simulink model "SIL_Raspi_control_panel"  (R2018b)
settings: Solver=VariableStepAuto  StartTime=0.0  StopTime=30  RelTol=1e-3  EnableMultiTasking=on
values from neighbouring files (symbols this model uses):
  INTAB1 = INTAB{1}    [MVP4.m]
  INTAB3 = INTAB{3}    [MVP4.m]
  INTAB4 = zeros(length(height), 6)    [MVP4.m]
libraries: embdlinuxlib x2, raspberrypilib x1
settings Model: ExtModeTrigDuration=2  Creator=benkl  LastModifiedBy=benkl
settings SolverCC: PositivePriorityOrder=on  AutoInsertRateTranBlk=on
settings OptimizationCC: EnhancedBackFolding=on  PassReuseOutputArgsAs=Individual arguments  MaxStackSize=64  OptimizeBlockOrder=speed  DifferentSizesBufferReuse=on  OptimizationCustomize=off
settings DebuggingCC: ParameterTunabilityLossMsg=error
settings HardwareCC: ProdBitPerPointer=32  ProdBitPerSizeT=32  ProdBitPerPtrDiffT=32  ProdLargestAtomicInteger=Long  ProdLargestAtomicFloat=Double  ProdWordSize=32  ProdHWDeviceType=ARM Compatible->ARM Cortex
settings SFSimCC: MATLABDynamicMemAlloc=off
settings RTWCC: SystemTargetFile=ert.tlc  HardwareBoard=Raspberry Pi  TLCOptions="-aInlineSetEventsForThisBaseRateFcn=TLC_FALSE -aSuppressMultiTaskScheduler=TLC_FALSE  -aRateBasedStepFcn=0"  TemplateMakefile=ert_default_tmf  Toolchain=GNU GCC Raspberry Pi  BuildConfiguration=Faster Runs  IncludeHyperlinkInReport=on
settings CodeAppCC: ForceParamTrailComments=on  IgnoreCustomStorageClasses=off  OperatorAnnotations=on  SimulinkDataObjDesc=on  SFDataObjDesc=on  InsertBlockDesc=on
settings ERTTargetCC: SupportContinuousTime=on  SupportVariableSizeSignals=on  ExtMode=on  ExtModeMexArgs='192.168.137.74' 0 17725

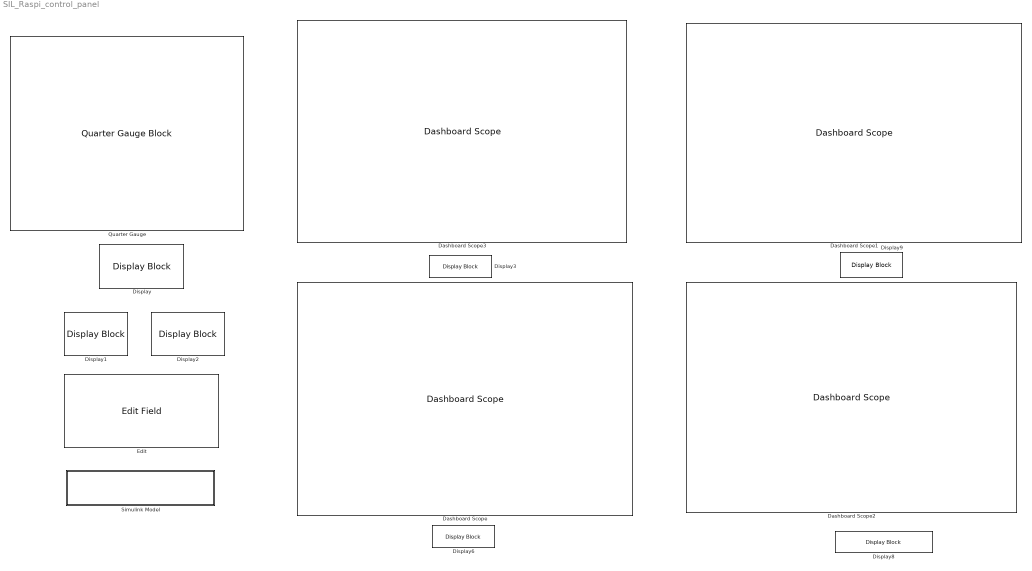
== system SIL_Raspi_control_panel ==
  Dashboard Scope : DashboardScope  WebBlockId=367  Ymin=0  Ymax=400
  Dashboard Scope1 : DashboardScope  WebBlockId=368  Ymin=0  Ymax=4000
  Dashboard Scope2 : DashboardScope  WebBlockId=406  Ymin=0.0030000000000000001  Ymax=0.01  ScaleAtStop=off
  Dashboard Scope3 : DashboardScope  WebBlockId=376  Ymin=-0.5  Ymax=0.5  ScaleAtStop=off
  Display : DisplayBlock  WebBlockId=375
  Display1 : DisplayBlock  WebBlockId=377
  Display2 : DisplayBlock  WebBlockId=379
  Display3 : DisplayBlock  WebBlockId=390  LabelPosition=Hide
  Display6 : DisplayBlock  WebBlockId=393  LabelPosition=Hide
  Display8 : DisplayBlock  WebBlockId=395  LabelPosition=Hide
  Display9 : DisplayBlock  WebBlockId=396  LabelPosition=Hide
  Edit : EditField  WebBlockId=389  ShowInitialText=on  Alignment=Center
  Quarter Gauge : QuarterGaugeBlock  WebBlockId=374  ScaleMax=77
  Simulink Model : Subsystem

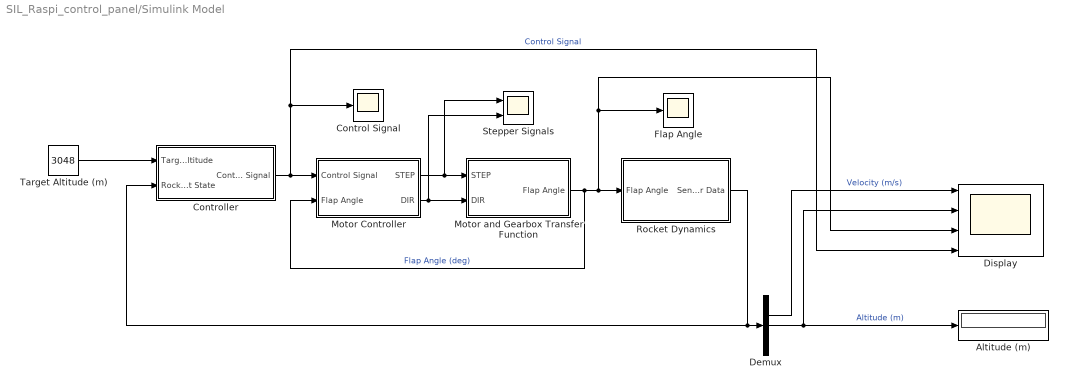
== system SIL_Raspi_control_panel/Simulink Model ==
  Altitude (m) : Display
  Control Signal : Scope
  Controller : Subsystem
  Demux : Demux  Outputs=5
  Display : Scope  NumInputPorts=4
  Flap Angle : Scope
  Motor Controller : Subsystem
  Motor and Gearbox Transfer Function : Subsystem
  Rocket Dynamics : Subsystem
  Stepper Signals : Scope  NumInputPorts=2
  "Target Altitude (m) " : Constant  Value=3048
  wires:
  Rocket Dynamics/1(Sensor Data) -> Demux/1, Controller/2(Rocket State)
  Motor and Gearbox Transfer Function/1(Flap Angle) -> Motor Controller/2(Flap Angle), Rocket Dynamics/1(Flap Angle), Display/3, Flap Angle/1  "Flap Angle (deg)"
  "Target Altitude (m) "/1 -> Controller/1(Target Altitude)
  Controller/1(Control Signal) -> Display/4, Control Signal/1, Motor Controller/1(Control Signal)  "Control Signal"
  Motor Controller/2(DIR) -> Stepper Signals/2, Motor and Gearbox Transfer Function/2(DIR)
  Motor Controller/1(STEP) -> Stepper Signals/1, Motor and Gearbox Transfer Function/1(STEP)
  Demux/2 -> Display/1  "Velocity (m/s)"
  Demux/3 -> Altitude (m)/1, Display/2  "Altitude (m)"

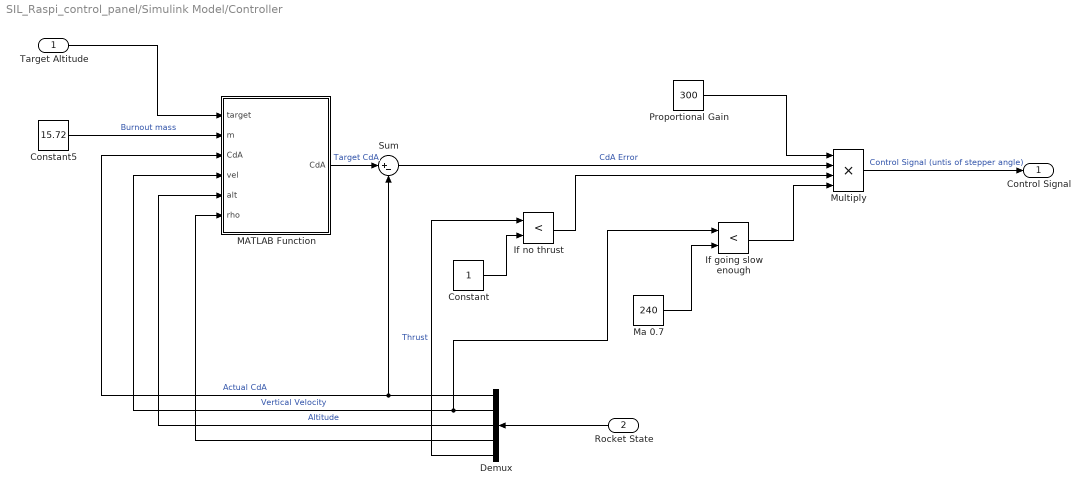
== system SIL_Raspi_control_panel/Simulink Model/Controller ==
  Target Altitude : Inport
  Rocket State : Inport  Port=2
  Constant : Constant
  Constant5 : Constant  Value=15.72
  Demux : Demux  Outputs=5
  If going slow enough : RelationalOperator  Operator=<  OutDataTypeStr=boolean  RndMeth=Simplest
  If no thrust : RelationalOperator  Operator=<  OutDataTypeStr=boolean  RndMeth=Simplest
  MATLAB Function : MATLAB Function  TreatAsAtomicUnit=on
  Ma 0.7 : Constant  Value=240
  Multiply : Product  Inputs=4
  Proportional Gain : Constant  Value=300
  Sum : Sum  Inputs=|+-
  Control Signal : Outport
  wires:
  Proportional Gain/1 -> Multiply/1
  Constant5/1 -> MATLAB Function/2(m)  "Burnout mass"
  Multiply/1 -> Control Signal/1  "Control Signal (untis of stepper angle)"
  MATLAB Function/1(CdA) -> Sum/1  "Target CdA"
  Sum/1 -> Multiply/2  "CdA Error"
  Demux/5 -> If no thrust/1  "Thrust"
  Rocket State/1 -> Demux/1
  Demux/3 -> MATLAB Function/5(alt)  "Altitude"
  Demux/2 -> If going slow enough/1, MATLAB Function/4(vel)  "Vertical Velocity"
  Demux/4 -> MATLAB Function/6(rho)
  Target Altitude/1 -> MATLAB Function/1(target)
  Demux/1 -> Sum/2, MATLAB Function/3("CdA ")  "Actual CdA"
  If no thrust/1 -> Multiply/3
  Constant/1 -> If no thrust/2
  If going slow enough/1 -> Multiply/4
  Ma 0.7/1 -> If going slow enough/2

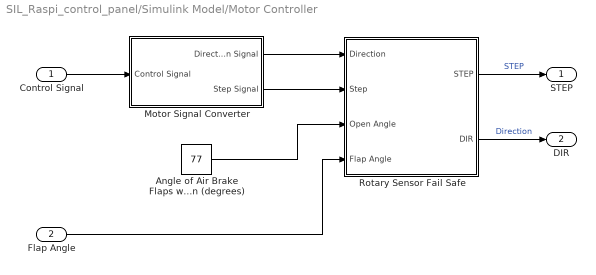
== system SIL_Raspi_control_panel/Simulink Model/Motor Controller ==
  Control Signal : Inport
  Flap Angle : Inport  Port=2
  Angle of Air Brake Flaps when Fully Open (degrees) : Constant  Value=77
  Motor Signal Converter : Subsystem
  Rotary Sensor Fail Safe : Subsystem
  STEP : Outport
  DIR : Outport  Port=2
  wires:
  Control Signal/1 -> Motor Signal Converter/1(Control Signal)
  Motor Signal Converter/2(Step Signal) -> Rotary Sensor Fail Safe/2(Step)
  Motor Signal Converter/1(Direction Signal) -> Rotary Sensor Fail Safe/1(Direction)
  Angle of Air Brake Flaps when Fully Open (degrees)/1 -> Rotary Sensor Fail Safe/3(Open Angle)
  Rotary Sensor Fail Safe/1(STEP) -> STEP/1  "STEP"
  Flap Angle/1 -> Rotary Sensor Fail Safe/4(Flap Angle)
  Rotary Sensor Fail Safe/2(DIR) -> DIR/1  "Direction"

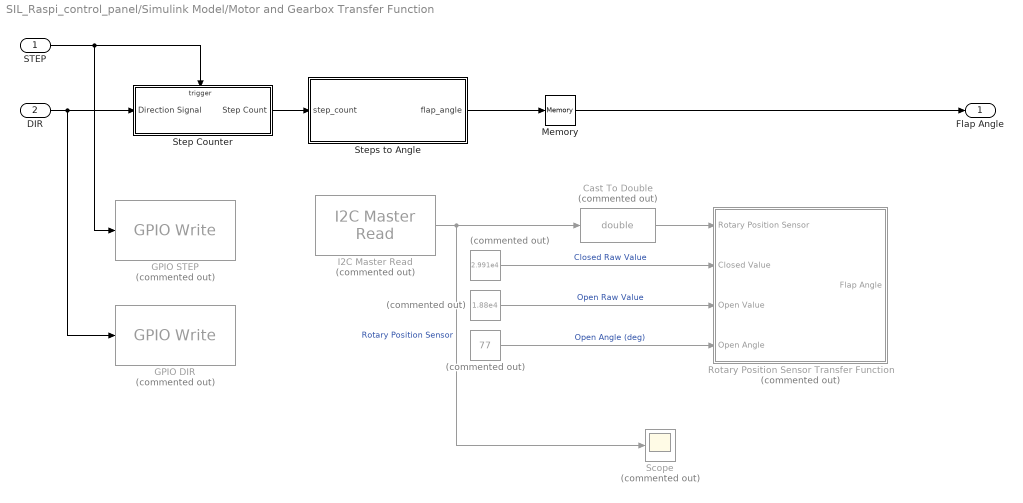
== system SIL_Raspi_control_panel/Simulink Model/Motor and Gearbox Transfer Function ==
  STEP : Inport
  DIR : Inport  Port=2
  " " : Constant  Commented=on  Value=2.991e4
  "  " : Constant  Commented=on  Value=77
  " " : Constant  Commented=on  Value=1.88e4
  Cast To Double : DataTypeConversion  Commented=on  OutDataTypeStr=double
  GPIO DIR : embdlinuxlib/GPIO Write  Commented=on  board=Model B+  gpio=21  direction=Output  blockPlatform=Raspberry Pi
      settings: SourceProductName=Simulink Support Package for Raspberry Pi Hardware  SourceProductBaseCode=RASPPI
  GPIO STEP : embdlinuxlib/GPIO Write  Commented=on  board=Model B+  gpio=20  direction=Output  blockPlatform=Raspberry Pi
      settings: SourceProductName=Simulink Support Package for Raspberry Pi Hardware  SourceProductBaseCode=RASPPI
  I2C Master Read : raspberrypilib/I2C Master Read  Commented=on  BoardProperty=Pi 3 Model B+  Mode=Master  SlaveAddress=72  SlaveByteOrder=BigEndian  Direction=Receiver  RegisterAddressMode=on  RegisterAddress=0  SlaveDataType=int16  DataLength=1  NoAck=off  RepeatedStart=off  OutputStatus=off  SampleTime=0.005
      settings: SourceProductName=Simulink Support Package for Raspberry Pi Hardware  SourceProductBaseCode=RASPPI
  Memory : Memory
  Rotary Position Sensor Transfer Function : Subsystem  Commented=on
  Scope : Scope  Commented=on
  Step Counter : Subsystem
  Steps to Angle : MATLAB Function  TreatAsAtomicUnit=on
  Flap Angle : Outport
  wires:
  Step Counter/1(Step Count) -> Steps to Angle/1(step_count)
  Steps to Angle/1(flap_angle) -> Memory/1
  "  "/1 -> Rotary Position Sensor Transfer Function/4(Open Angle)  "Open Angle (deg)"
  I2C Master Read/1 -> Scope/1, Cast To Double/1  "Rotary Position Sensor"
  " "/1 -> Rotary Position Sensor Transfer Function/2(Closed Value)  "Closed Raw Value"
  " "/1 -> Rotary Position Sensor Transfer Function/3(Open Value)  "Open Raw Value"
  STEP/1 -> GPIO STEP/1, Step Counter/Trigger
  DIR/1 -> GPIO DIR/1, Step Counter/1(Direction Signal)
  Cast To Double/1 -> Rotary Position Sensor Transfer Function/1(Rotary Position Sensor)
  Memory/1 -> Flap Angle/1

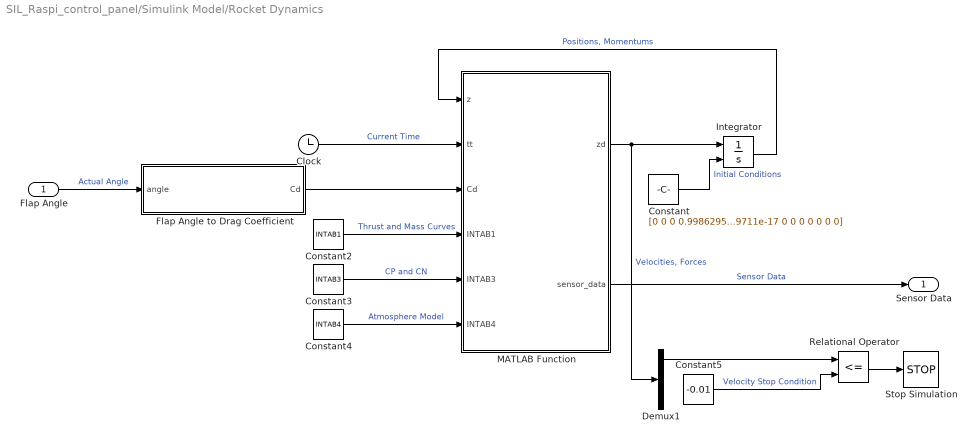
== system SIL_Raspi_control_panel/Simulink Model/Rocket Dynamics ==
  Flap Angle : Inport
  Clock : Clock
  Constant : Constant  Value="[0\t0\t0\t0.998629534754574\t-0.0523359562429438\t1.92279183879711e-17\t0\t0\t0\t0\t0\t0\t0]"
  Constant2 : Constant  Value=INTAB1  VectorParams1D=off
  Constant3 : Constant  Value=INTAB3  VectorParams1D=off
  Constant4 : Constant  Value=INTAB4  VectorParams1D=off
  Constant5 : Constant  Value=-0.01
  Demux1 : Demux  Outputs=13
  Flap Angle to Drag Coefficient : MATLAB Function  TreatAsAtomicUnit=on
  Integrator : Integrator  InitialConditionSource=external
  MATLAB Function : MATLAB Function  TreatAsAtomicUnit=on
  Relational Operator : RelationalOperator  Operator=<=  OutDataTypeStr=boolean  RndMeth=Simplest
  Stop Simulation : Stop
  Sensor Data : Outport
  wires:
  Clock/1 -> MATLAB Function/2(tt)  "Current Time"
  Integrator/1 -> MATLAB Function/1(z)  "Positions, Momentums"
  Constant4/1 -> MATLAB Function/6(INTAB4)  "Atmosphere Model"
  MATLAB Function/1(zd) -> Integrator/1, Demux1/1  "Velocities, Forces"
  Constant5/1 -> Relational Operator/2  "Velocity Stop Condition"
  Constant3/1 -> MATLAB Function/5(INTAB3)  "CP and CN"
  Constant2/1 -> MATLAB Function/4(INTAB1)  "Thrust and Mass Curves"
  MATLAB Function/2(sensor_data) -> Sensor Data/1  "Sensor Data"
  Flap Angle/1 -> Flap Angle to Drag Coefficient/1(angle)  "Actual Angle"
  Flap Angle to Drag Coefficient/1(Cd) -> MATLAB Function/3(Cd)
  Relational Operator/1 -> Stop Simulation/1
  Constant/1 -> Integrator/2  "Initial Conditions"
  Demux1/3 -> Relational Operator/1

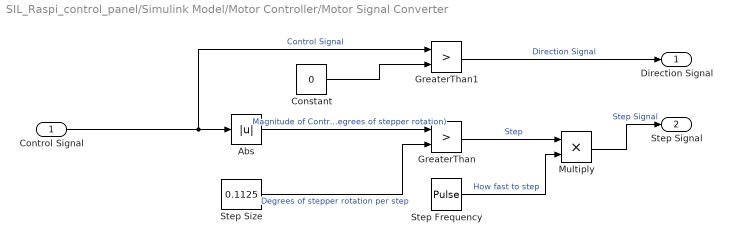
== system SIL_Raspi_control_panel/Simulink Model/Motor Controller/Motor Signal Converter ==
  Control Signal : Inport
  Abs : Abs
  Constant : Constant  Value=0
  GreaterThan : RelationalOperator  Operator=>  OutDataTypeStr=boolean  RndMeth=Simplest
  GreaterThan1 : RelationalOperator  Operator=>  OutDataTypeStr=boolean  RndMeth=Simplest
  Multiply : Product
  Step Frequency : DiscretePulseGenerator  PulseType=Time based  Period=0.005  PulseWidth=50
  Step Size : Constant  Value=0.1125
  Direction Signal : Outport
  Step Signal : Outport  Port=2
  wires:
  Abs/1 -> GreaterThan/1  "Magnitude of Control Signal (degrees of stepper rotation)"
  Constant/1 -> GreaterThan1/2
  Step Size/1 -> GreaterThan/2  "Degrees of stepper rotation per step"
  Control Signal/1 -> GreaterThan1/1, Abs/1  "Control Signal"
  Step Frequency/1 -> Multiply/2  "How fast to step"
  GreaterThan/1 -> Multiply/1  "Step"
  Multiply/1 -> Step Signal/1  "Step Signal"
  GreaterThan1/1 -> Direction Signal/1  "Direction Signal"

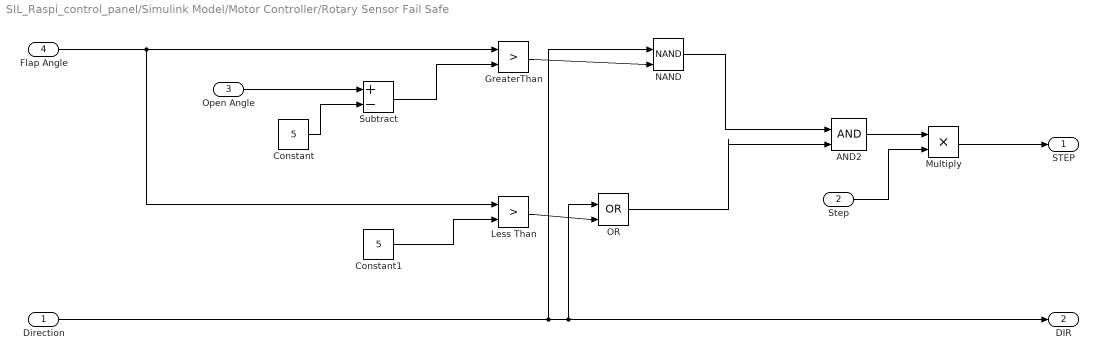
== system SIL_Raspi_control_panel/Simulink Model/Motor Controller/Rotary Sensor Fail Safe ==
  Direction : Inport
  Step : Inport  Port=2
  Open Angle : Inport  Port=3
  Flap Angle : Inport  Port=4
  AND2 : Logic  IconShape=distinctive  AllPortsSameDT=off  OutDataTypeStr=boolean
  Constant : Constant  Value=5
  Constant1 : Constant  Value=5
  GreaterThan : RelationalOperator  Operator=>  OutDataTypeStr=boolean  RndMeth=Simplest
  Less Than : RelationalOperator  Operator=>  OutDataTypeStr=boolean  RndMeth=Simplest
  Multiply : Product
  NAND : Logic  Operator=NAND  IconShape=distinctive  AllPortsSameDT=off  OutDataTypeStr=boolean
  OR : Logic  Operator=OR  IconShape=distinctive  AllPortsSameDT=off  OutDataTypeStr=boolean
  Subtract : Sum  Inputs=+-
  STEP : Outport
  DIR : Outport  Port=2
  wires:
  Flap Angle/1 -> Less Than/1, GreaterThan/1
  Constant/1 -> Subtract/2
  Open Angle/1 -> Subtract/1
  Subtract/1 -> GreaterThan/2
  GreaterThan/1 -> NAND/2
  Multiply/1 -> STEP/1
  Step/1 -> Multiply/2
  Direction/1 -> NAND/1, OR/1, DIR/1
  AND2/1 -> Multiply/1
  Less Than/1 -> OR/2
  Constant1/1 -> Less Than/2
  OR/1 -> AND2/2
  NAND/1 -> AND2/1

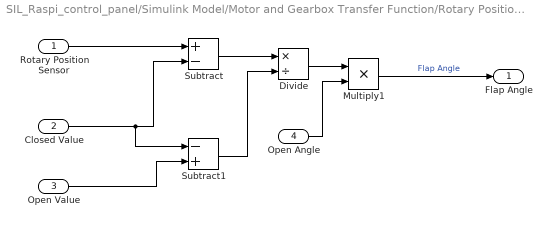
== system SIL_Raspi_control_panel/Simulink Model/Motor and Gearbox Transfer Function/Rotary Position Sensor Transfer Function ==
  Rotary Position Sensor : Inport
  Closed Value : Inport  Port=2
  Open Value : Inport  Port=3
  Open Angle : Inport  Port=4
  Divide : Product  Inputs=*/
  Multiply1 : Product
  Subtract : Sum  Inputs=+-
  Subtract1 : Sum  Inputs=-+
  Flap Angle : Outport
  wires:
  Subtract/1 -> Divide/1
  Closed Value/1 -> Subtract1/1, Subtract/2
  Divide/1 -> Multiply1/1
  Open Angle/1 -> Multiply1/2
  Subtract1/1 -> Divide/2
  Rotary Position Sensor/1 -> Subtract/1
  Open Value/1 -> Subtract1/2
  Multiply1/1 -> Flap Angle/1  "Flap Angle"

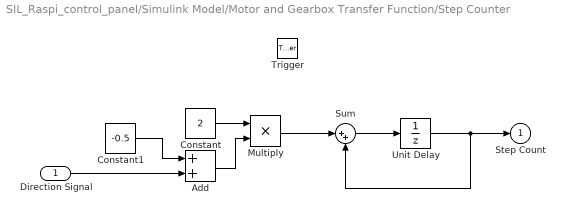
== system SIL_Raspi_control_panel/Simulink Model/Motor and Gearbox Transfer Function/Step Counter ==
  Direction Signal : Inport
  Trigger : TriggerPort  VariantControl=Variant  PortDimensions=1
  Add : Sum
  Constant : Constant  Value=2
  Constant1 : Constant  Value=-0.5
  Multiply : Product
  Sum : Sum  Inputs=|++  SaturateOnIntegerOverflow=on  InputSameDT=on  OutDataTypeStr=Inherit: Same as first input
  Unit Delay : UnitDelay  SampleTime=-1
  Step Count : Outport  InitialOutput=0
  wires:
  Direction Signal/1 -> Add/2
  Add/1 -> Multiply/2
  Constant1/1 -> Add/1
  Constant/1 -> Multiply/1
  Sum/1 -> Unit Delay/1
  Unit Delay/1 -> Step Count/1, Sum/2
  Multiply/1 -> Sum/1

== matlab function SIL_Raspi_control_panel/Simulink Model/Controller/MATLAB Function ==
  data: target input; m input; CdA output; CdA input; vel input; alt input; rho input
function CdA  = drag_predictor(target, m, CdA, vel, alt, rho)
%DRAG_PREDICTOR calculates the optimal drag coefficient based on current state

a = m/(rho*0.9); % bit of hard-coding jank to get the prediction more acurate
b = 2*9.81/vel^2;
c = target - alt;
CdA_opt = (-a*Lambert_W((-b*c*exp(-b*c)),-1)-a*b*c)/c; % Closed form solved in matlab

if isreal(CdA_opt) && ~isnan(CdA_opt)
%     if CdA_opt > 0.001 && CdA_opt < 0.01 % Set upper and lower bounds on CdA (m^2)
%         CdA = CdA_opt;
%     elseif CdA_opt < 0.001
%         CdA = 0.001;
%     else 
%         CdA = 0.01;
%     end
%     
    CdA = CdA_opt;
end

if alt > target % If already too high, put brakes on as much as possible
    CdA = 1;
end

    function w = Lambert_W(x,branch)
        % Lambert_W  Functional inverse of x = w*exp(w).
        % w = Lambert_W(x), same as Lambert_W(x,0)
        % w = Lambert_W(x,0)  Primary or upper branch, W_0(x)
        % w = Lambert_W(x,-1)  Lower branch, W_{-1}(x)
        %
        % See: https://blogs.mathworks.com/cleve/2013/09/02/the-lambert-w-function/

        % Copyright 2013 The MathWorks, Inc.

        % Effective starting guess
        if nargin < 2 || branch ~= -1
           w = ones(size(x));  % Start above -1
        else  
           w = -2*ones(size(x));  % Start below -1
        end
        v = inf*w;
        
        
        % Haley's method
        ii = 0;
        while any(abs(w - v)./abs(w) > 1.e-6) && ii<1000
           v = w;
           e = exp(w);
           f = w.*e - x;  % Iterate to make this quantity zero
           w = w - f./((e.*(w+1) - (w+2).*f./(2*w+2)));
           ii = ii+1;
        end
    end

% in.alt = alt; % [m] rocket's current altitude
% in.vel = vel; % [m/s] rocket's current velocity
% in.rho = rho; % [kg/m^3] density of air
% in.m = m; % [kg] mass of rocket after burnout
% 
% % options = optimset('TolX', 1e-7);
% % [CdA_opt,~,exitflag] = fzero(@apogeeerror, CdA, options);
% % 
% % if exitflag==1
% %     CdA = CdA_opt;
% % end
% % 
% % 
% % 
% %     function apogee = apogeeerror(CdA) % Finds the difference between the estimated and actual apogee
% %         x = log( complex(CdA*rho/(2*m*9.81)*vel^2 + 1) );
% %         if isreal(x)
% %             apogee = alt + m/(CdA*rho) * x - target;
% %         else
% %             apogee = 1e9;
% %         end
% %     end
% 
% % 
% % try
%     CdA_opt = secant(@apogeeerror, CdA, in); % Might want to use a more robust solver in the future
%     if CdA_opt > 0.001 && CdA_opt < 0.01 % Set upper and lower bounds on CdA (m^2)
%         CdA = CdA_opt;
%     end % Otherwise keep estimated term for CdA
% % catch
% % end
% %     
% 
%     function [x] = secant(fun, x1, in)
%     %SECANT is a zero-finding function based on the secant method
%     %   'fun' is the function handle for which the zero is desired
%     %   'x1' is the initial guess
%     %   'in' is a struct containing any additional inputs 'fun' might require
%     %   'x' is the value of the zero
%         x_eps = x1*0.005; % Set the tolerance to be 0.5% of initial guess
%         x2 = x1-x1*0.01; % Set a second point 1% away from the original guess
%         F1 = fun(x1, in); % Evaluate function at x1
%         F2 = fun(x2, in); % Evaluate function at x2
%         
%         
%         
%         kk = 1; % Set up counter
%         kk_max = 100;
%         while abs(x2-x1)>=x_eps && kk<kk_max % While error is too large and counter is less than max
%             x3 = x2 - F2*(x2-x1)/(F2-F1);
%             x1 = x2; % Move everything forward
%             x2 = x3;
%             F1 = F2;
%             F2 = fun(x2, in);
%             if ~isreal(F2) % If non-real
%                 x = NaN;
%                 return
%             end
%             kk = kk+1;
%         end
%         x = x2;
%     end
% 
%     function apogee = apogeeerror(CdA, in) % Finds the difference between the estimated and actual apogee
% %         if CdA*in.rho/(2*in.m*9.81) * in.vel^2 + 1 <= 0
% %             sup = 0;
% %         end
%         apogee = in.alt + in.m/(CdA*in.rho) * log( complex(CdA*in.rho/(2*in.m*9.81) * in.vel^2 + 1) ) - target;
%     end

end

== matlab function SIL_Raspi_control_panel/Simulink Model/Motor and Gearbox Transfer Function/Steps to Angle ==
  data: step_count input; flap_angle output
function flap_angle = Steps_to_Angle_TF(step_count)
% Calulates the flap angle based on the stepper commands
%   Will be replaced by physical system in prototype

GR = 2.5; % Gear ratio between stepper and flap
step_size = 0.1125; % [degrees] angle of one step of the stepper

flap_angle = step_count*step_size*GR;

== matlab function SIL_Raspi_control_panel/Simulink Model/Rocket Dynamics/Flap Angle to Drag Coefficient ==
  data: angle input; Cd output
function Cd = dragTF(angle) % Angle is the flap angle (as sensed by position sensor)

%%%%%%%%%%%%%% REPLACE THIS WITH BETTER MODEL BASED ON CFD %%%%%%%%%%%%%%%%
% Also add mach number dependency

Cd_rocket = 0.4; % Coefficient of drag of rocket
A_ref = 0.010751315458748; % [m^2] rocket reference area
Cd_flat_plate = 1.1; % From CFD

A_flat_plate = -3.953e-7*angle^2 + 8.737e-5*angle + 4.547e-5; % Calculate exposed area (quadratic fit from solidworks angle-area points)
Cd = Cd_rocket + Cd_flat_plate*A_flat_plate/A_ref; % Calculate Drag Coefficient

== matlab function SIL_Raspi_control_panel/Simulink Model/Rocket Dynamics/MATLAB Function ==
  data: z input; tt input; zd output; Cd input; INTAB1 input; INTAB3 input; INTAB4 input; sensor_data output
function [zd,sensor_data]=blastoff6dof(z,tt,Cd,INTAB1,INTAB3,INTAB4)
% % Constants **************************************************************
% RL=4.3; % Launch rail length
% Ar=0.010751315458748; % Rocket aerodynamic reference area
% 
% 
% % Unpack z ***************************************************************
% zn=z(1); % Postion vector
% Pz=z(2); % Translational momentum vector
% 
% % Gravity ****************************************************************
% g=6.6742E-11*5.9742E24/(6378100+zn)^2;
% 
% 
% % EXTRACT DATA FROM INPUT TABLES 1, 3, and 4 *****************************
% % INTAB1 *****************************************************************
% t=INTAB1(:,1); % Get time data from input table
% if tt<=t(1)
%     Ti = INTAB1(1,2);
%     Mi = INTAB1(1,3);
% elseif tt<t(end) % If time is within bounds of array
%     for ii = 2:length(t)
%         if tt <= t(ii) % Find first index that is larger than OF
%             break
%         end
%     end
%     T = INTAB1(:,2);
%     Ti = (tt-t(ii-1))/(t(ii)-t(ii-1))*(T(ii)-T(ii-1)) + T(ii); % Thrust-time data
%     M = INTAB1(:,3);
%     Mi = (tt-t(ii-1))/(t(ii)-t(ii-1))*(M(ii)-M(ii-1)) + M(ii); % Mass-time data
% else
%     Ti=INTAB1(end,2);
%     Mi=INTAB1(end,3);
% end
% 
% % INTAB4 *****************************************************************
% ztb=INTAB4(:,1); %Get altitude data from input table
% if zn<ztb(end) && zn>=ztb(1)
%     for ii = 2:length(ztb)
%         if zn <= ztb(ii) % Find first index that is larger than OF
%             break
%         end
%     end
%     RHO = INTAB4(:,5);
%     rho = (zn-ztb(ii-1))/(ztb(ii)-ztb(ii-1))*(RHO(ii)-RHO(ii-1)) + RHO(ii); % Atmospheric density
%     TEMP = INTAB4(:,5);
%     temp = (zn-ztb(ii-1))/(ztb(ii)-ztb(ii-1))*(TEMP(ii)-TEMP(ii-1)) + TEMP(ii); % Atmospheric temperature
%     Pressure = 287*rho*temp;%Atmospheric Pressure
% else % If outside of table bounds
%     temp=(-131.21+(0.00299*zn))+273.15; % Random atmosphere model???
%     Pressure=0.002488*(temp/216.6)^-11.388;
%     rho=Pressure/287*temp;
% end
% 
% 
% % Rocket Velocity Calculations *******************************************
% Vz=Pz./Mi; % Rocket earth relative velocity vector
% 
% % Force vector calculations **********************************************
% FA=Cd*0.5*rho*(Vz^2)*Ar; % Calculate axial aerodynamic force
% mg=Mi*g; % Gravity
% 
% % Output calculations ****************************************************
% % Calculate position derivatives (velocities relative to earth)
% zdot=Vz;
% 
% % Calculate translational momentum derivatives (forces)
% if Ti<=mg && zn<0.1 % If thrust is smaller than gravity and flight just began
%     Fz=0;
% else
%     Fz=Ti-FA-mg; % Z Force vector component
% end
% 
% %ODE output
% zd=zeros(2,1);
% zd(1)=zdot;
% zd(2)=Fz;
% 
% % Sensor output **********************************************************
% sensor_data=zeros(5,1);
% sensor_data(1) = Cd*Ar; % CdA
% sensor_data(2) = zdot; % Vertical Velocity
% sensor_data(3) = zn; % Altitude
% sensor_data(4) = rho; % Air Density
% sensor_data(5) = Ti; % Thrust
% 
% 
% Constants **************************************************************
RL=4.3; % Launch rail length
Ar=0.010751315458748; % Rocket aerodynamic reference area


% Unpack z ***************************************************************
xn=z(1); % Postion vector
yn=z(2); % "
zn=z(3); % "
s=z(4); % Quaternion scalar
vx=z(5); % Quaternion vector
vy=z(6); % "
vz=z(7); % "
Px=z(8); % Translational momentum vector
Py=z(9); % "
Pz=z(10); % "
Ltheta=z(11); % Rotational momentum vector
Lphi=z(12); % "
Lpsi=z(13); % "

xt=[xn;yn;zn]; % Rocket position vector
qt=[s vx vy vz]; % Rocket quaternion
Pt=[Px;Py;Pz]; % Rocket translational momentum vector
Lt=[Ltheta;Lphi;Lpsi]; % Rocket rotational momentum vector


% Gravity ****************************************************************
g=6.6742E-11*5.9742E24/(6378100+zn)^2;


% EXTRACT DATA FROM INPUT TABLES 1, 3, and 4 *****************************
% INTAB1 *****************************************************************
t=INTAB1(:,1); % Get time data from input table
if tt<=t(1)
    Ti=INTAB1(1,2);
    Mi=INTAB1(1,3);
    Ixxi=INTAB1(1,4);
    Iyyi=INTAB1(1,5);
    Izzi=INTAB1(1,6);
    Ixyi=INTAB1(1,7);
    Ixzi=INTAB1(1,8);
    Iyzi=INTAB1(1,9);
    Xcmi=INTAB1(1,10);
    Cda1=INTAB1(1,11);
elseif tt<t(end) && tt>=t(1) % If time is within bounds of array
    Ti=interp1(t,INTAB1(:,2),tt); % Thrust-time data
    Mi=interp1(t,INTAB1(:,3),tt); % Mass-time data
    Ixxi=interp1(t,INTAB1(:,4),tt); % Moments of inertia-time data
    Iyyi=interp1(t,INTAB1(:,5),tt); % "
    Izzi=interp1(t,INTAB1(:,6),tt); % "
    Ixyi=interp1(t,INTAB1(:,7),tt); % Products of inertia-time data
    Ixzi=interp1(t,INTAB1(:,8),tt); % "
    Iyzi=interp1(t,INTAB1(:,9),tt); % "
    Xcmi=interp1(t,INTAB1(:,10),tt); % Center of mass-time data
    Cda1=interp1(t,INTAB1(:,11),tt); % Thrust damping moment coefficient
else
    Ti=INTAB1(end,2);
    Mi=INTAB1(end,3);
    Ixxi=INTAB1(end,4);
    Iyyi=INTAB1(end,5);
    Izzi=INTAB1(end,6);
    Ixyi=INTAB1(end,7);
    Ixzi=INTAB1(end,8);
    Iyzi=INTAB1(end,9);
    Xcmi=INTAB1(end,10);
    Cda1=INTAB1(end,11);
end
Ibody=[Ixxi Ixyi Ixzi;Ixyi Iyyi Iyzi;Ixzi Iyzi Izzi]; % Inertia tensor

% INTAB3 *****************************************************************
Cn=INTAB3(1);
Cp=INTAB3(2);

% INTAB4 *****************************************************************
ztb=INTAB4(:,1); %Get altitude data from input table
if zn<ztb(end) && zn>=ztb(1)
    Wxi=interp1(ztb,INTAB4(:,2),zn);%Wind velocity vector
    Wyi=interp1(ztb,INTAB4(:,3),zn);%"
    Wzi=interp1(ztb,INTAB4(:,4),zn);%"
    
    rho=interp1(ztb,INTAB4(:,5),zn);%Atmospheric density
    temp=interp1(ztb,INTAB4(:,6),zn);%Atmospheric Temperature
    Pressure = 287*rho*temp;%Atmospheric Pressure
else % If outside of table bounds
    Wxi=INTAB4(end,2);%Wind velocity vector
    Wyi=INTAB4(end,3);%"
    Wzi=INTAB4(end,4);%"
    
    temp=(-131.21+(0.00299*zn))+273.15; % Random atmosphere model???
    Pressure=0.002488*(temp/216.6)^-11.388;
    rho=Pressure/287*temp;
end


% Rocket Velocity Calculations *******************************************
if vectormag(xt)<=RL % While vehicle is still on the launch rail
    Wt=[0;0;0];
else
    Wt=[Wxi;Wyi;Wzi]; % Wind vector
end
Ut=Pt./Mi; % Rocket earth relative velocity vector
Vt=Ut+Wt; % Rocket atmosphere relative velocity vector


% Rocket orientation calculations ****************************************
qt=vectornorm(qt); % Normalise quaternion
s=qt(1); % Quaternion scalar part only
vt=[qt(2);qt(3);qt(4)]; % Quaternion vector part only
Rt=quaternion_to_matrix(qt); % Transform quaternion to rotation matrix
RA=Rt*[0;0;1]; % Roll axis vector


% Center of pressure velocity calculations *******************************
Xbar=Cp-Xcmi; % Moment arm
Xbart=-Xbar*RA; % Moment arm vector

It = Rt*Ibody*Rt'; % Inertia tensor in global coordinates
omegat=It\Lt; % Angular velocity vector

Vcpt=Vt+cross(omegat, Xbart); % Velocity vector of center of pressure
Vcptmag=vectormag(Vcpt); % Magnitude of velocity of center of pressure
Vcptnorm=vectornorm(Vcpt); % Direction of velocity of center of pressure

if Vcptmag==0 % Set angle of attack to zero if not moving
    alphacp=0;
else
    dprod=dot(Vcptnorm,RA); % Dot product of velocity and rocket axis
    if dprod>1
        dprod=1;
    end
    alphacp=acos(dprod); % Angle of attack
end


% Force vector calculations **********************************************
FA=Cd*0.5*rho*(Vcptmag^2)*Ar*cos(alphacp); % Calculate axial aerodynamic force
FAt=FA*-RA; % Axial drag vector

FNcp=Cn*alphacp*0.5*rho*(Vcptmag^2)*Ar*sin(alphacp); % Calculate normal aerodynamic force
momaxcp=cross(RA,Vcptnorm); % axis of pitching motion
momaxcp=vectornorm(momaxcp);
FNn=cross(RA,momaxcp);
FNn=vectornorm(FNn); % Direction of normal force
FNt=FNcp*FNn; % Normal force vector

Tt=Ti*RA; % Thrust Vector

mg=Mi*g; % Gravity

% Torque vector calculations *********************************************
Tqf=(FNcp*Xbar)*momaxcp; % Aerodynamic torque due to normal force
Tqm=-Cda1*omegat; % Thrust damping torque
% Tqm=(-Cda1*omega)*omegaax2; % Thrust damping torque
Tqt=Tqf+Tqm; % Total torque on rocket


% Output calculations ****************************************************
% Calculate position derivatives (velocities relative to earth)
xdot=Ut(1);
ydot=Ut(2);
zdot=Ut(3);

% Calculate quaternion derivative
sdot=(-dot(omegat,vt))*0.5;
vtdot=((s*omegat)+(cross(omegat,vt)))*0.5;
vxdot=vtdot(1);
vydot=vtdot(2);
vzdot=vtdot(3);

% Calculate translational momentum derivatives (forces)
if Ti<=mg && zn<0.1 % If thrust is smaller than gravity and flight just began
    Fx=0;
    Fy=0;
    Fz=0;
else
    Fx=Tt(1)+FAt(1)+FNt(1); % X Force vector component
    Fy=Tt(2)+FAt(2)+FNt(2); % Y Force vector component
    Fz=Tt(3)+FAt(3)+FNt(3)-mg; % Z Force vector component
end

% Calculate rotational momentum derivatives (torques)
if vectormag(xt)<=RL % While still on launch rail
    Ttheta=0;
    Tphi=0;
    Tpsi=0;
else
    Ttheta=Tqt(1); % Torque vector
    Tphi=Tqt(2); %"
    Tpsi=Tqt(3); %"
end

%ODE output
zd=zeros(13,1);
zd(1)=xdot;
zd(2)=ydot;
zd(3)=zdot;
zd(4)=sdot;
zd(5)=vxdot;
zd(6)=vydot;
zd(7)=vzdot;
zd(8)=Fx;
zd(9)=Fy;
zd(10)=Fz;
zd(11)=Ttheta;
zd(12)=Tphi;
zd(13)=Tpsi;

if Vcptmag > 500
    g = 9;
end

% Sensor output **********************************************************
sensor_data=zeros(5,1);
sensor_data(1) = Cd*Ar; % CdA
sensor_data(2) = zdot; % Vertical Velocity
sensor_data(3) = zn; % Altitude
sensor_data(4) = rho; % Air Density
sensor_data(5) = Ti; % Thrust

% function [zd,sensor_data]=blastoff6dof(z,tt,Cd,INTAB1,INTAB3,INTAB4)
% 
% % Constants **************************************************************
% RL=4.3; % Launch rail length
% Ar=0.010751315458748; % Rocket aerodynamic reference area
% 
% 
% % Unpack z ***************************************************************
% xn=z(1); % Postion vector
% yn=z(2); % "
% zn=z(3); % "
% s=z(4); % Quaternion scalar
% vx=z(5); % Quaternion vector
% vy=z(6); % "
% vz=z(7); % "
% Px=z(8); % Translational momentum vector
% Py=z(9); % "
% Pz=z(10); % "
% Ltheta=z(11); % Rotational momentum vector
% Lphi=z(12); % "
% Lpsi=z(13); % "
% 
% xt=[xn;yn;zn]; % Rocket position vector
% qt=[s vx vy vz]; % Rocket quaternion
% Pt=[Px;Py;Pz]; % Rocket translational momentum vector
% Lt=[Ltheta;Lphi;Lpsi]; % Rocket rotational momentum vector
% 
% 
% % Gravity ****************************************************************
% g=6.6742E-11*5.9742E24/(6378100+zn)^2;
% 
% 
% % EXTRACT DATA FROM INPUT TABLES 1, 3, and 4 *****************************
% % INTAB1 *****************************************************************
% t=INTAB1(:,1); % Get time data from input table
% if tt<=t(1)
%     Ti=INTAB1(1,2);
%     Mi=INTAB1(1,3);
%     Ixxi=INTAB1(1,4);
%     Iyyi=INTAB1(1,5);
%     Izzi=INTAB1(1,6);
%     Ixyi=INTAB1(1,7);
%     Ixzi=INTAB1(1,8);
%     Iyzi=INTAB1(1,9);
%     Xcmi=INTAB1(1,10);
%     Cda1=INTAB1(1,11);
% elseif tt<t(end) && tt>=t(1) % If time is within bounds of array
%     Ti=interp1(t,INTAB1(:,2),tt); % Thrust-time data
%     Mi=interp1(t,INTAB1(:,3),tt); % Mass-time data
%     Ixxi=interp1(t,INTAB1(:,4),tt); % Moments of inertia-time data
%     Iyyi=interp1(t,INTAB1(:,5),tt); % "
%     Izzi=interp1(t,INTAB1(:,6),tt); % "
%     Ixyi=interp1(t,INTAB1(:,7),tt); % Products of inertia-time data
%     Ixzi=interp1(t,INTAB1(:,8),tt); % "
%     Iyzi=interp1(t,INTAB1(:,9),tt); % "
%     Xcmi=interp1(t,INTAB1(:,10),tt); % Center of mass-time data
%     Cda1=interp1(t,INTAB1(:,11),tt); % Thrust damping moment coefficient
% else
%     Ti=INTAB1(end,2);
%     Mi=INTAB1(end,3);
%     Ixxi=INTAB1(end,4);
%     Iyyi=INTAB1(end,5);
%     Izzi=INTAB1(end,6);
%     Ixyi=INTAB1(end,7);
%     Ixzi=INTAB1(end,8);
%     Iyzi=INTAB1(end,9);
%     Xcmi=INTAB1(end,10);
%     Cda1=INTAB1(end,11);
% end
% Ibody=[Ixxi Ixyi Ixzi;Ixyi Iyyi Iyzi;Ixzi Iyzi Izzi]; % Inertia tensor
% 
% % INTAB3 *****************************************************************
% Cn=INTAB3(1);
% Cp=INTAB3(2);
% 
% % INTAB4 *****************************************************************
% ztb=INTAB4(:,1); %Get altitude data from input table
% if zn<ztb(end) && zn>=ztb(1)
%     Wxi=interp1(ztb,INTAB4(:,2),zn);%Wind velocity vector
%     Wyi=interp1(ztb,INTAB4(:,3),zn);%"
%     Wzi=interp1(ztb,INTAB4(:,4),zn);%"
%     
%     rho=interp1(ztb,INTAB4(:,5),zn);%Atmospheric density
%     temp=interp1(ztb,INTAB4(:,6),zn);%Atmospheric Temperature
%     Pressure = 287*rho*temp;%Atmospheric Pressure
% else % If outside of table bounds
%     Wxi=INTAB4(end,2);%Wind velocity vector
%     Wyi=INTAB4(end,3);%"
%     Wzi=INTAB4(end,4);%"
%     
%     temp=(-131.21+(0.00299*zn))+273.15; % Random atmosphere model???
%     Pressure=0.002488*(temp/216.6)^-11.388;
%     rho=Pressure/287*temp;
% end
% 
% 
% % Rocket Velocity Calculations *******************************************
% if vectormag(xt)<=RL % While vehicle is still on the launch rail
%     Wt=[0;0;0];
% else
%     Wt=[Wxi;Wyi;Wzi]; % Wind vector
% end
% Ut=Pt./Mi; % Rocket earth relative velocity vector
% Vt=Ut+Wt; % Rocket atmosphere relative velocity vector
% 
% 
% % Rocket orientation calculations ****************************************
% qt=vectornorm(qt); % Normalise quaternion
% s=qt(1); % Quaternion scalar part only
% vt=[qt(2);qt(3);qt(4)]; % Quaternion vector part only
% Rt=quaternion_to_matrix(qt); % Transform quaternion to rotation matrix
% RA=Rt*[0;0;1]; % Roll axis vector
% 
% 
% % Center of pressure velocity calculations *******************************
% Xbar=Cp-Xcmi; % Moment arm
% Xbart=-Xbar*RA; % Moment arm vector
% 
% It = Rt*Ibody*Rt'; % Inertia tensor in global coordinates
% omegat=It\Lt; % Angular velocity vector
% 
% Vcpt=Vt+cross(omegat, Xbart); % Velocity vector of center of pressure
% Vcptmag=vectormag(Vcpt); % Magnitude of velocity of center of pressure
% Vcptnorm=vectornorm(Vcpt); % Direction of velocity of center of pressure
% 
% if Vcptmag==0 % Set angle of attack to zero if not moving
%     alphacp=0;
% else
%     dprod=dot(Vcptnorm,RA); % Dot product of velocity and rocket axis
%     if dprod>1
%         dprod=1;
%     end
%     alphacp=acos(dprod); % Angle of attack
% end
% 
% 
% % Force vector calculations **********************************************
% FA=Cd*0.5*rho*(Vcptmag^2)*Ar*cos(alphacp); % Calculate axial aerodynamic force
% FAt=FA*-RA; % Axial drag vector
% 
% FNcp=Cn*alphacp*0.5*rho*(Vcptmag^2)*Ar*sin(alphacp); % Calculate normal aerodynamic force
% momaxcp=cross(RA,Vcptnorm); % axis of pitching motion
% momaxcp=vectornorm(momaxcp);
% FNn=cross(RA,momaxcp);
% FNn=vectornorm(FNn); % Direction of normal force
% FNt=FNcp*FNn; % Normal force vector
% 
% Tt=Ti*RA; % Thrust Vector
% 
% mg=Mi*g; % Gravity
% 
% % Torque vector calculations *********************************************
% Tqf=(FNcp*Xbar)*momaxcp; % Aerodynamic torque due to normal force
% Tqm=-Cda1*omegat; % Thrust damping torque
% % Tqm=(-Cda1*omega)*omegaax2; % Thrust damping torque
% Tqt=Tqf+Tqm; % Total torque on rocket
% 
% 
% % Output calculations ****************************************************
% % Calculate position derivatives (velocities relative to earth)
% xdot=Ut(1);
% ydot=Ut(2);
% zdot=Ut(3);
% 
% % Calculate quaternion derivative
% sdot=(-dot(omegat,vt))*0.5;
% vtdot=((s*omegat)+(cross(omegat,vt)))*0.5;
% vxdot=vtdot(1);
% vydot=vtdot(2);
% vzdot=vtdot(3);
% 
% % Calculate translational momentum derivatives (forces)
% if Ti<=mg && zn<0.1 % If thrust is smaller than gravity and flight just began
%     Fx=0;
%     Fy=0;
%     Fz=0;
% else
%     Fx=Tt(1)+FAt(1)+FNt(1); % X Force vector component
%     Fy=Tt(2)+FAt(2)+FNt(2); % Y Force vector component
%     Fz=Tt(3)+FAt(3)+FNt(3)-mg; % Z Force vector component
% end
% 
% % Calculate rotational momentum derivatives (torques)
% if vectormag(xt)<=RL % While still on launch rail
%     Ttheta=0;
%     Tphi=0;
%     Tpsi=0;
% else
%     Ttheta=Tqt(1); % Torque vector
%     Tphi=Tqt(2); %"
%     Tpsi=Tqt(3); %"
% end
% 
% %ODE output
% zd=zeros(13,1);
% zd(1)=xdot;
% zd(2)=ydot;
% zd(3)=zdot;
% zd(4)=sdot;
% zd(5)=vxdot;
% zd(6)=vydot;
% zd(7)=vzdot;
% zd(8)=Fx;
% zd(9)=Fy;
% zd(10)=Fz;
% zd(11)=Ttheta;
% zd(12)=Tphi;
% zd(13)=Tpsi;
% 
% % Sensor output **********************************************************
% sensor_data=zeros(5,1);
% sensor_data(1) = Cd*Ar; % CdA
% sensor_data(2) = zdot; % Vertical Velocity
% sensor_data(3) = zn; % Altitude
% sensor_data(4) = rho; % Air Density
% sensor_data(5) = Ti; % Thrust

end
